simulink model "state"  (R2021a)
settings: Solver=ode5  StartTime=0.0  StopTime=40  MaxStep=0.001  RelTol=1e-3  EnableMultiTasking=on
values from neighbouring files (symbols this model uses):
  A_down = double(subs(A_sym, [X; u], [X_down; u_eq]))    [my_real_pendulum.m]
  A_up = double(subs(A_sym, [X; u], [X_up; u_eq]))    [my_real_pendulum.m]
  B_down = double(subs(B_sym, [X; u], [X_down; u_eq]))    [my_real_pendulum.m]
  B_up = double(subs(B_sym, [X; u], [X_up; u_eq]))    [my_real_pendulum.m]
  C = [0 1 0 0 ... (first row only)    [my_real_pendulum.m]
  K_I_down = K_sloz_down(5)    [my_real_pendulum.m]
  K_I_up = K_sloz_up(5)    [my_real_pendulum.m]
  K_new_down = K_sloz_down(1:4)    [my_real_pendulum.m]
  K_new_up = K_sloz_up(1:4)    [my_real_pendulum.m]
  L_down = place(A_down', C', p_poz_down)'    [my_real_pendulum.m]
  L_up = place(A_up', C', p_poz_up)'    [my_real_pendulum.m]
undefined symbols (not defined in the file or in its folder): Humusoft, MF624
libraries: sldrtlib x3
settings Model: Creator=fuka  LastModifiedBy=koubajac
settings SolverCC: AlgebraicLoopSolver=TrustRegion
settings DataIOCC: LimitDataPoints=on  SaveFormat=Array  SignalLoggingSaveFormat=ModelDataLogs  ReturnWorkspaceOutputs=off
settings OptimizationCC: ExpressionDepthLimit=2147483647  InitFltsAndDblsToZero=on
settings DebuggingCC: SaveWithParameterizedLinksMsg=none  UnderspecifiedInitializationDetection=Classic  MergeDetectMultiDrivingBlocksExec=none  SignalResolutionControl=TryResolveAllWithWarning  SolverPrmCheckMsg=warning  MultiTaskDSMMsg=warning  MultiTaskCondExecSysMsg=none  FcnCallInpInsideContextMsg=warning  StateNameClashWarn=warning  SFUnexpectedBacktrackingDiag=warning  SFNoUnconditionalDefaultTransitionDiag=warning  SFExecutionAtInitializationDiag=none  SFMachineParentedDataDiag=warning  ArithmeticOperatorsInVariantConditions=warning
settings ModelReferenceCC: PropagateSignalLabelsOutOfModel=off
settings SFSimCC: SimUseLocalCustomCode=off  CustomCodeUndefinedFunction=UseInterfaceOnly
settings RTWCC: Description=Simulink Desktop Real-Time  SystemTargetFile=sldrt.tlc  TemplateMakefile=sldrt.tmf  RTWUseLocalCustomCode=off  RTWCompilerOptimization=on
settings CodeAppCC: MaxIdLength=95  StateflowObjectComments=on
settings SimulinkDesktopRealTimeCC: TargetPreCompLibLocation=C:\MATLAB\R2021a\toolbox\sldrt\lib\win64  TargetLangStandard=C89/C90 (ANSI)
settings ConfigComp: CovMetricSettings=dw  CovSaveCumulativeToWorkspaceVar=on  CovSaveSingleToWorkspaceVar=on  CovExternalEMLEnable=off  CovSFcnEnable=off

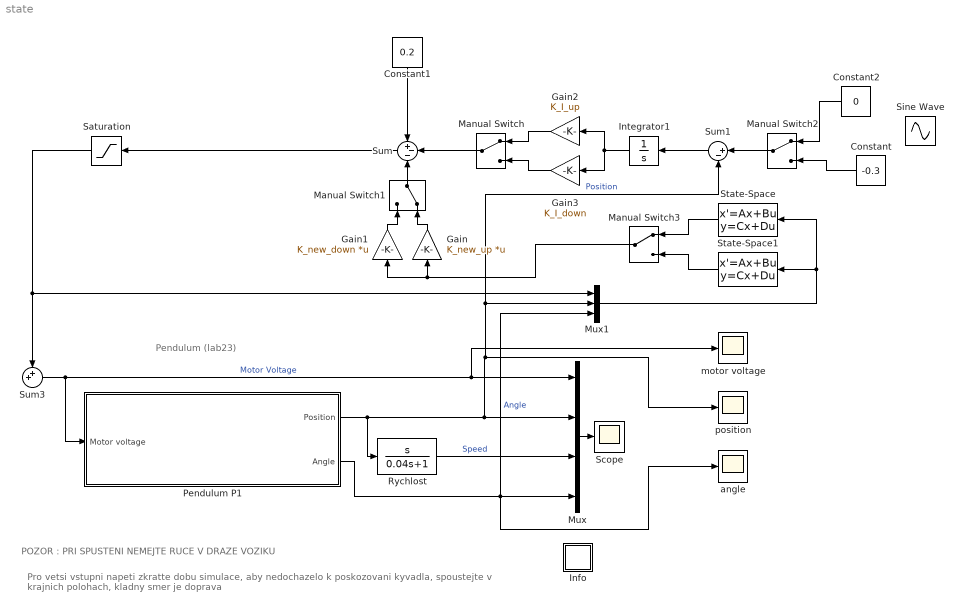
== system state ==
  note: POZOR : PRI SPUSTENI NEMEJTE RUCE V DRAZE VOZIKU
  note: Pro vetsi vstupni napeti zkratte dobu simulace, aby nedochazelo k poskozovani
      |  kyvadla, spoustejte v krajnich polohach, kladny smer je doprava
  note: Pendulum (lab23)
  Constant : Constant  Value=-0.3
  Constant1 : Constant  Value=0.2
  Constant2 : Constant  Value=0
  Gain : Gain  Gain=K_new_up  Multiplication=Matrix(K*u)
  Gain1 : Gain  Gain=K_new_down  Multiplication=Matrix(K*u)
  Gain2 : Gain  Gain=K_I_up
  Gain3 : Gain  Gain=K_I_down
  Info : Subsystem
      mask Display: disp('?')
  Integrator1 : Integrator
  Manual Switch : ManualSwitch
  Manual Switch1 : ManualSwitch  CurrentSetting=0
  Manual Switch2 : ManualSwitch
  Manual Switch3 : ManualSwitch
  Mux : Mux
  Mux1 : Mux  Inputs=3
  Pendulum P1 : Subsystem  InitFcn=warning off;  mask(Pendulum P1 in laboratory K23){Ts=0.001}
      mask prompts: Ts "Sampling time  {Ts = 0.001 s;   0.001 - 0.01 s}"
      mask help: Pendulum P1 in laboratory K23 - Real Time Communication
      mask Help:
      | Servo AMIRA S1, S4 in laboratory K23, K26 - Real Time Communication. <br><br>
      | 
      | This is a model of the Servomechanism, which is composed of two identical motors (motor and generator) connected together with solid motor shaft. First motor is used as a generator - it can be used to simulation of a varying  moment of inertia. The second motor takes control of the rotational speed of the servomechanism or the angle of turning of the motor shaft.<br>
      | 
      | There are two inputs and three outputs in the model. Inputs are voltages of generator and motor.
      | Outputs are speed of the servomechanism, the angle of turning of the motor shaft and current of the motor.<br><br>
      | In Simulink, the signals are normalized.
      mask Display: image(imread('P1pic.tif'))
  Rychlost : TransferFcn  Numerator=[1 0]  Denominator=[0.04 1]
  Saturation : Saturate  UpperLimit=1  LowerLimit=-1
  Scope : Scope
  Sine Wave : Sin  Amplitude=0.2  Frequency=0.5  SampleTime=0
  State-Space : StateSpace  A=A_up-L_up*C  B=[B_up, L_up]  C=eye(4)  D=zeros(4,3)  InitialCondition=0
  State-Space1 : StateSpace  A=A_down-L_down*C  B=[B_down, L_down]  C=eye(4)  D=zeros(4,3)  InitialCondition=0
  Sum : Sum  Inputs=+--
  Sum1 : Sum  Inputs=|+-
  Sum3 : Sum  Inputs=++|
  angle : Scope
  motor voltage : Scope
  position : Scope
  wires:
  Mux/1 -> Scope/1
  Pendulum P1/1(Position) -> Rychlost/1, position/1, Sum1/2, Mux1/2, Mux/2  "Position"
  Rychlost/1 -> Mux/3  "Speed"
  Pendulum P1/2(Angle) -> Mux1/3, Mux/4, angle/1  "Angle"
  Sum3/1 -> motor voltage/1, Mux/1, Pendulum P1/1(Motor voltage)  "Motor Voltage"
  Saturation/1 -> Mux1/1, Sum3/1
  Sum/1 -> Saturation/1
  Manual Switch/1 -> Sum/2
  Manual Switch1/1 -> Sum/3
  Gain/1 -> Manual Switch1/2
  Gain1/1 -> Manual Switch1/1
  Gain2/1 -> Manual Switch/1
  Gain3/1 -> Manual Switch/2
  Integrator1/1 -> Gain3/1, Gain2/1
  Sum1/1 -> Integrator1/1
  Manual Switch2/1 -> Sum1/1
  Constant/1 -> Manual Switch2/2
  Manual Switch3/1 -> Gain/1, Gain1/1
  State-Space/1 -> Manual Switch3/1
  State-Space1/1 -> Manual Switch3/2
  Mux1/1 -> State-Space/1, State-Space1/1
  Constant1/1 -> Sum/1
  Constant2/1 -> Manual Switch2/1

== system state/Info ==
  note: Urceno pro mereni prechodovych charakteristik realneho systemu inverzni kyvadlo.
      |  Periodu vzorkovani Ts volte v rozsahu 0.0005 s < Ts < 0.001 s  (dop. Ts = 0.001 s).
  note: Vozik presunte do leve krajni polohy. Po spusteni simulace dojede k prave krajni
      | poloze. Presunte jej ke koncovemu spinaci a zmente znamenko zesileni. Vozik
      | se vrati do vychozi polohy. Pri vetsim vstupnim napeti zkratte dobu simulace!!!
  note: Umisteni voziku
  note: Merena data jsou ukladana po radcich do matice ty v pracovnim prostoru Matlabu.
      | Prvni sloupec matice ty predstavuje cas a dalsi pak jednotlive promenne v poradi
      | vstupu do bloku multiplexoru osciloskopu. Krome toho je jeste k dispozici samotny
      | vektor casu tout. Prubehy velicin zobrazite napr. prikazem: plot(ty(:,1),ty(:,2:4)).
  note: Nezapomente si ulozit namerena data napr. prikazem: save <jmeno> ty
  note: Ve formatu ASCII je pak ulozite prikazem: save <jmeno> ty -ascii
  note: C: J.Fuka 2007-2015 pro Matlab 2014b s RTWT
  note: Kyvadlo P1 (lab. 23)

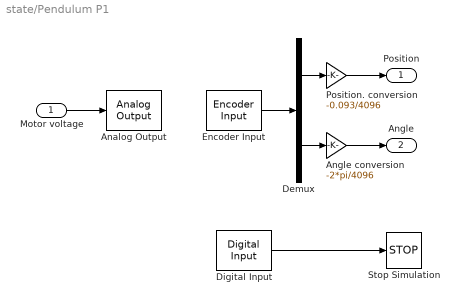
== system state/Pendulum P1 ==
  Motor voltage : Inport
  Analog Output : sldrtlib/Analog Output  SampleTime=Ts  MaxMissedTicks=200  ShowMissedTicks=off  YieldWhenWaiting=on  DrvName=Humusoft/MF624  DrvAddress=4294967295  DrvOptions=0  Channels=1  RangeMode=2  VoltRange=1  InitialValue=0  FinalValue=0
      settings: AttributesFormatString=Humusoft\nMF624 [auto]
  Angle conversion : Gain  Gain=-2*pi/4096
  Demux : Demux  Outputs=2
      settings: DisplayOption=none
  Digital Input : sldrtlib/Digital Input  SampleTime=0.005  MaxMissedTicks=100  ShowMissedTicks=off  YieldWhenWaiting=off  DrvName=Humusoft/MF624  DrvAddress=4294967295  DrvOptions=0  Channels=3  BitMode=1  DataType=9
      settings: AttributesFormatString=Humusoft\nMF624 [auto]  SourceProductBaseCode=WT
  Encoder Input : sldrtlib/Encoder Input  SampleTime=Ts  MaxMissedTicks=200  ShowMissedTicks=off  YieldWhenWaiting=on  DrvName=Humusoft/MF624  DrvAddress=4294967295  DrvOptions=0  Channels=[1 2]  QuadMode=3  IndexPulse=2  InputFilter=Inf  DataType=1
      settings: AttributesFormatString=Humusoft\nMF624 [auto]
  Position. conversion : Gain  Gain=-0.093/4096
  Stop Simulation : Stop
  Position : Outport
  Angle : Outport  Port=2
  wires:
  Position. conversion/1 -> Position/1
  Demux/2 -> Angle conversion/1
  Angle conversion/1 -> Angle/1
  Encoder Input/1 -> Demux/1
  Demux/1 -> Position. conversion/1
  Digital Input/1 -> Stop Simulation/1
  Motor voltage/1 -> Analog Output/1
